simulink library "Drivetrain_Library"  (R2020b)
settings: Solver=VariableStepAuto  StartTime=0.0  StopTime=10.0  RelTol=1e-3
undefined symbols (not defined in the file or in its folder): MotorLeft, MotorRight
libraries: simulink x18, mbd_s32k1xx_ec_toolbox x8
(part 2 of 2)

== stateflow chart Drivetrain_Library/UQM Control Logic (R)/Drive Train ==
  state Drive_Mode [parallel]
    entry:
    universal_cmd_cnt = 0;
    during:
    universal_cmd_cnt = mod(universal_cmd_cnt,16);
    settings: executionOrder=5
    state Normal
      entry:
      output_chart_state = 3;
      during:
      % setting bits 0-3 to torque mode and bits 4-7 to the counter value
      output_universal_cmd(1) = bitor(uint8(1),bitshift(universal_cmd_cnt,4));
      output_universal_cmd(2) = bitor(bitshift(uint8(1),4),bitshift(uint8(input_flag_F),3));
      output_universal_cmd(3:4) = convert_val_to_UQM_CAN_bytes(input_torque_request,-350,350,0.1,3212.8);
      output_universal_cmd(5:6) = convert_val_to_UQM_CAN_bytes(input_velocity_limit_forward,0,5400,0.5,16064);
      output_universal_cmd(7:8) = convert_val_to_UQM_CAN_bytes(input_velocity_limit_reverse,-900,0,0.5,16064);
    state LimitedTorque_LimpHome
      entry:
      output_chart_state = 2;
      % limit what goes out on universal command, override them
      during:
      % setting bits 0-3 to torque mode and bits 4-7 to the counter value
      output_universal_cmd(1) = bitor(uint8(1),bitshift(universal_cmd_cnt,4));
      output_universal_cmd(2) = bitor(bitshift(uint8(1),4),bitshift(uint8(input_flag_F),3));
      output_universal_cmd(3:4) = convert_val_to_UQM_CAN_bytes(input_torque_request,-100,100,0.1,3212.8);
      output_universal_cmd(5:6) = convert_val_to_UQM_CAN_bytes(input_velocity_limit_forward,0,900,0.5,16064);
      output_universal_cmd(7:8) = convert_val_to_UQM_CAN_bytes(input_velocity_limit_reverse,-900,0,0.5,16064);
    state ZeroTorque_Startup
      entry:
      output_chart_state = 1;
      % sending universal command msg (torque/speed limits)
      % completely override for command w zero torque
      during:
      % setting universal command to coast
      output_universal_cmd = uint8([0; 8; hex2dec('80'); hex2dec('7D'); ...
      hex2dec('80'); hex2dec('7D'); hex2dec('80'); hex2dec('7D')]);
      % setting bits 0-3 to torque mode and bits 4-7 to the counter value
      output_universal_cmd(1) = bitor(uint8(1),bitshift(universal_cmd_cnt,4));
    state Shutdown
      entry:
      output_chart_state = 0;
      during:
      % setting universal command to coast
      output_universal_cmd = uint8([0; 8; hex2dec('80'); hex2dec('7D'); ...
      hex2dec('80'); hex2dec('7D'); hex2dec('80'); hex2dec('7D')]);
      % setting bits 0-3 to torque mode and bits 4-7 to the counter value
      output_universal_cmd(1) = bitor(uint8(1),bitshift(universal_cmd_cnt,4));
    Normal -> Shutdown [commented out] : CAN_WD_Timeout
    ZeroTorque_Startup -> Normal [order 3] : [1==input_brake_switch && ...
        | (xor(input_flag_F, input_flag_R)) && ...
        | 1==output_comms_good_self && ...
        | 1==input_comms_good_other && ...
        | 3==input_steering_mode && ...
        | FNR_velocity_match_flag==1 && ...
        | (input_torque_request>-25 && input_torque_request<5)]
        | % negative side might need to be bigger
    Normal -> Shutdown [order 1] : inputs_outside_range
    Normal -> ZeroTorque_Startup [order 3] : [FNR_velocity_match_flag==0]
    Normal -> ZeroTorque_Startup [order 4] : [input_steering_mode==0 || ...
        | input_steering_mode==1]
    Normal -> ZeroTorque_Startup [order 2] : [input_flag_F==0 && ...
        | input_flag_R==0]
    Normal -> LimitedTorque_LimpHome [order 5] : [2==input_steering_mode]
    LimitedTorque_LimpHome -> Normal [order 3] : [1==output_comms_good_self && ...
        | 1==input_comms_good_other && ...
        | 3==input_steering_mode && ...
        | FNR_velocity_match_flag==1 && ...
        | (input_torque_request>-100 && input_torque_request<100)]
        | % negative side might need to be bigger
    LimitedTorque_LimpHome -> Shutdown [commented out] : CAN_WD_Timeout
    LimitedTorque_LimpHome -> Shutdown [order 1] : inputs_outside_range
    LimitedTorque_LimpHome -> ZeroTorque_Startup [order 2] : [(input_flag_F==0 && ...
        | input_flag_R==0) || ...
        | 1==input_steering_mode || ...
        | 0==input_steering_mode]
    ZeroTorque_Startup -> LimitedTorque_LimpHome [order 1] : [1==input_brake_switch && ...
        | (xor(input_flag_F, input_flag_R)) && ...
        | ( ((0==output_comms_good_self && 1==input_comms_good_other) || (1==output_comms_good_self && 0==input_comms_good_other)) || ...
        | (1==output_comms_good_self && 1==input_comms_good_other && 2==input_steering_mode && FNR_velocity_match_flag==1) ) && ...
        | (input_torque_request>-25 && input_torque_request<5)]
        | % negative side might need to be bigger
    (default) -> ZeroTorque_Startup
    ZeroTorque_Startup -> Shutdown [commented out] : CAN_WD_Timeout
    ZeroTorque_Startup -> Shutdown [order 2] : inputs_outside_range
  state Fault_Lamp_Control [parallel]
    settings: executionOrder=6
    state Steady_OFF
      during:
      output_fault_lamp = false;
    state Blink_OFF
      during:
      output_fault_lamp = false;
    state Blink_ON
      during:
      output_fault_lamp = true;
    state Steady_ON
      during:
      output_fault_lamp = true;
    Steady_OFF -> Fault_Lamp_Control : [output_chart_state ~= 3]
    (junction 149) -> Steady_OFF [order 2] : [output_chart_state == 3]
    Blink_ON -> Steady_OFF [order 1] : [output_chart_state == 3]
    Blink_OFF -> Steady_OFF [order 1] : [output_chart_state == 3]
    Blink_OFF -> Blink_ON [order 3] : [elapsed > output_chart_state*0.4]
    (default) -> (junction 149)
    (junction 149) -> Blink_ON [order 3]
    (junction 149) -> Steady_ON [order 1] : [output_chart_state == 0]
    Blink_ON -> Blink_OFF [order 3] : [elapsed > output_chart_state*0.4]
    Blink_ON -> Steady_ON [order 2] : [output_chart_state == 0]
    Blink_OFF -> Steady_ON [order 2] : [output_chart_state == 0]
    Steady_ON -> Fault_Lamp_Control : [output_chart_state ~= 0]
  state CAN_Watchdog [parallel]
    entry:
    lastUQMWatchDogTime = 0;
    settings: executionOrder=1
    state CAN_Good
      entry:
      output_comms_good_self=true;
    state CAN_Lost
      entry:
      output_comms_good_self=false;
    (default) -> CAN_Good
    CAN_Good -> CAN_Watchdog [order 2] : [input_UQM_timeStamp ~= lastUQMWatchDogTime]{lastUQMWatchDogTime = input_UQM_timeStamp}
    CAN_Good -> CAN_Lost [order 1] : [elapsed > 1.2 && lastUQMWatchDogTime ~= 0] {send(CAN_WD_Timeout, Drive_Mode)}
  state Input_check [parallel]
    during:
    settings: executionOrder=4
    state Input_check_if_statement
      (default) -> (junction 279)
      (junction 279) -> (junction 280) [order 1] : [input_velocity_limit_forward>5400 || ...
          | input_velocity_limit_forward<0]
      (junction 279) -> (junction 266) [order 2]
      (junction 280) -> (junction 281)
      (junction 266) -> (junction 269) [order 1] : [input_velocity_limit_reverse<0 || ...
          | input_velocity_limit_reverse>900]
      (junction 266) -> (junction 265) [order 2]
      (junction 269) -> (junction 268)
      (junction 265) -> (junction 270) [order 1] : [input_torque_request>350 || ...
          | input_torque_request<-350]
      (junction 265) -> (junction 179) [order 2]
      (junction 270) -> (junction 267)
      (junction 179) -> (junction 180) [order 1] : [1==input_flag_F && 1==input_flag_R]
      (junction 179) -> (junction 181) [order 2]
      (junction 180) -> (junction 185)
      (junction 181) -> (junction 182) [order 1] : [input_accelerator_value < 1.4 || ...
          | input_accelerator_value > 4.5 ]
      (junction 181) -> (junction 183) [order 2]
      (junction 182) -> (junction 184)
      (junction 184) -> (junction 183) : {send(inputs_outside_range, Drive_Mode)}
      (junction 185) -> (junction 184)
      (junction 267) -> (junction 185)
      (junction 268) -> (junction 267)
      (junction 281) -> (junction 268)
      (junction 183) -> (junction 352)
    Input_check_if_statement -> Input_check
  state Fault_check [parallel]
    settings: executionOrder=2
    state Fault_check_if_statement
      (default) -> (junction 255)
      (junction 255) -> (junction 253) [order 1] : [bitand(input_UQM_status(7),uint8(hex2dec('21')))~=0]
      (junction 255) -> (junction 254) [order 2]
      (junction 253) -> (junction 251)
      (junction 254) -> (junction 252) [order 1] : [bitand(input_UQM_status(8),uint8(hex2dec('7E')))~=0]
      (junction 254) -> (junction 239) [order 2]
      (junction 252) -> (junction 250)
      (junction 239) -> (junction 240) [order 1] : [input_UQM_status(5)~=1]
      (junction 239) -> (junction 241) [order 2]
      (junction 240) -> (junction 248)
      (junction 241) -> (junction 242) [order 1] : [input_UQM_status(2)~=0]
      (junction 241) -> (junction 243) [order 2]
      (junction 242) -> (junction 247)
      (junction 243) -> (junction 244) [order 1] : [input_UQM_status(1)~=0]
      (junction 243) -> (junction 245) [order 2]
      (junction 244) -> (junction 246)
      (junction 251) -> (junction 250)
      (junction 250) -> (junction 248)
      (junction 246) -> (junction 245) : {send(FAULT_DETECTED, Drive_Mode)}
      (junction 247) -> (junction 246)
      (junction 248) -> (junction 247)
      (junction 245) -> (junction 249)
    Fault_check_if_statement -> Fault_check
  state FNR_Velocity_Match [parallel]
    settings: executionOrder=3
    state FNR_Velocity_Match_if_statement
      (default) -> (junction 319)
      (junction 319) -> (junction 320) [order 1] : [-5>input_speed && 1==input_flag_F]
      (junction 319) -> (junction 321) [order 2]
      (junction 320) -> (junction 325)
      (junction 321) -> (junction 322) [order 1] : [5<input_speed && 1==input_flag_R]
      (junction 321) -> (junction 323) [order 2] : {FNR_velocity_match_flag=1;}
      (junction 322) -> (junction 324)
      (junction 324) -> (junction 323) : {FNR_velocity_match_flag=0;}
      (junction 325) -> (junction 324)
      (junction 323) -> (junction 326)
    FNR_Velocity_Match_if_statement -> FNR_Velocity_Match
  data: real_val function_input; lower_lim function_input; upper_lim function_input; gain_val function_input; offset_val function_input; output_bytes function_output; input_brake_switch input; input_comms_good_other input; input_steering_mode input; input_speed input; output_chart_state output; input_accelerator_value input; output_fault_lamp output boolean; input_flag_F input; input_flag_R input; input_UQM_status input uint8 size=8; input_UQM_timeStamp input; input_torque_request input; input_velocity_limit_forward input; input_velocity_limit_reverse input; output_universal_cmd output uint8 size=8; lastUQMWatchDogTime local; universal_cmd_cnt local; FNR_velocity_match_flag local; output_comms_good_self output
  events: FAULT_DETECTED local FUNCTION_CALL_EVENT; inputs_outside_range local FUNCTION_CALL_EVENT; CAN_WD_Timeout local FUNCTION_CALL_EVENT
  function output_bytes = convert_val_to_UQM_CAN_bytes(real_val,lower_lim,upper_lim,gain_val,offset_val):
    | function output_bytes = convert_val_to_UQM_CAN_bytes(real_val,lower_lim,upper_lim,gain_val,offset_val)
    | % saturate the real value between the upper and lower limits
    | real_val = max(real_val,lower_lim);
    | real_val = min(real_val,upper_lim);
    | % convert real value to UQM representation value
    | CAN_val = (round(10*(real_val+offset_val))/10)/gain_val;
    | % cast to uint16 data type
    | CAN_val_int = cast(CAN_val,'uint16');
    | CAN_bytes = typecast(CAN_val_int,'uint8');
    | output_bytes = CAN_bytes(1:2);
    | end
